simulink model "vinayquadcopter298"  (R2013b)
settings: Solver=ode45  StartTime=0.0  StopTime=10  RelTol=1e-3  EnableMultiTasking=on
values from neighbouring files (symbols this model uses):
  b = 3.13*10^(-5)    (= 3.13e-05)    [vinayparameters.m]
  d = 7.5*10^(-7)    (= 7.5e-07)    [vinayparameters.m]
  g = 9.81    [vinayparameters.m]
  Ix = 7.5*10^(-3)    (= 0.0075)    [vinayparameters.m]
  Iy = 7.5*10^(-3)    (= 0.0075)    [vinayparameters.m]
  Iz = 1.3*10^(-2)    (= 0.013)    [vinayparameters.m]
  Jr = 6.5*10^(-5)    (= 6.5e-05)    [vinayparameters.m]
  kdp = 0.4    [vinayparameters.m]
  kdps = 0.4    [vinayparameters.m]
  kdt = 0.4    [vinayparameters.m]
  kdz = 20    [vinayparameters.m]
  kpp = 0.8    [vinayparameters.m]
  kpps = 1    [vinayparameters.m]
  kpt = 1.2    [vinayparameters.m]
  kpz = 100    [vinayparameters.m]
  l = 0.23    [vinayparameters.m]
  m = 0.65    [vinayparameters.m]
libraries: simulink x7
settings Model: Creator=lcoelab  LastModifiedBy=VINAY
settings DataIOCC: SignalLoggingSaveFormat=ModelDataLogs
settings OptimizationCC: SimCompilerOptimization=off
settings DebuggingCC: UnderspecifiedInitializationDetection=Simplified  MergeDetectMultiDrivingBlocksExec=error  MultiTaskDSMMsg=warning  MultiTaskCondExecSysMsg=none  FcnCallInpInsideContextMsg=error  FrameProcessingCompatibilityMsg=error  LibraryContextMissingDiagnostic=warning  SFExecutionAtInitializationDiag=none
settings HardwareCC: ProdBitPerSizeT=32  ProdBitPerPtrDiffT=32
settings RTWCC: RTWCompilerOptimization=off
settings CodeAppCC: StateflowObjectComments=on
settings GRTTargetCC: TargetLangStandard=C89/C90 (ANSI)  CodeReplacementLibrary=None  CPPClassGenCompliant=on
settings ConfigComp: CovMetricSettings=dw  CovHtmlReporting=on  CovSaveCumulativeToWorkspaceVar=on  CovSaveSingleToWorkspaceVar=on  CovExternalEMLEnable=off

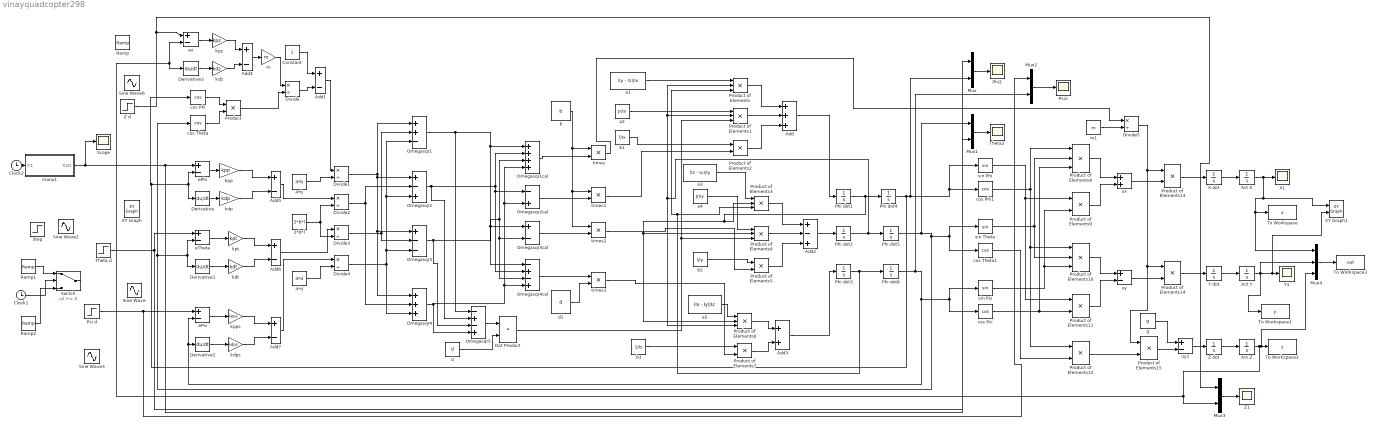
== system vinayquadcopter298 ==
  2*b*l : Constant  Value=2*b*l
  4*b : Constant  Value=4*b
  4*d : Constant  Value=4*d
  Act X : Integrator
  Act Y : Integrator
  Act Z : Integrator
  Add : Sum  Inputs=+++
  Add{1,4..7} (5 alike) : Sum  Inputs=+-
  Add2 : Sum  Inputs=+-+
  Add3 : Sum
  Clock1 : Clock
  Clock2 : Clock
  Constant : Constant
  Derivative{,1..3} (4 alike) : Derivative
  Divide{,1..5} (6 alike) : Product  Inputs=*/
  Dot Product : DotProduct  InputSameDT=on  OutDataTypeStr=Inherit: Inherit via internal rule
  Mux{,1..3} (4 alike) : Mux  Inputs=2
  Mux4 : Mux  Inputs=3
  Omegasqr1 : Sum  Inputs=++-
  Omegasqr1cal : Sum  Inputs=++++
  Omegasqr2 : Sum  Inputs=+-+
  Omegasqr2cal : Sum  Inputs=-+
  Omegasqr3 : Sum  Inputs=+--
  Omegasqr3cal : Sum  Inputs=+-
  Omegasqr4 : Sum  Inputs=+++
  Omegasqr4cal : Sum  Inputs=-+-+
  Omegasqr5 : Sum  Inputs=-+-+
  Phi dot1 : Integrator
  Phi dot{2..6} (5 alike) : Integrator  ZeroCross=off
  Phi2 : Scope
  Product : Product  RndMeth=Zero
  Product of Elements{,1,3..4,6,8,10} (7 alike) : Product  Inputs=3
  Product of Elements{2,5,7,9,11..15} (9 alike) : Product
  Psi d : Step  Time=0  After=0  SampleTime=0
  Psi2 : Scope
  Ramp : simulink/Sources/Ramp  slope=1  start=0  X0=0
  Ramp1 : simulink/Sources/Ramp  slope=0.1  start=0  X0=0
  Ramp2 : simulink/Sources/Ramp  slope=-0.1  start=0  X0=0
  Scope : Scope
  Sine Wave : Sin  Amplitude=10  Frequency=0.005*(2*pi)  Phase=pi/2  SampleTime=0
  Sine Wave2 : Sin  Amplitude=10  Frequency=0.005*(2*pi)  SampleTime=0
  Sine Wave3 : Sin  SampleTime=0
  Sine Wave6 : Sin  Amplitude=0  Frequency=0  SampleTime=0
  Step : Step  Time=0  After=5  SampleTime=0
  Switch : Switch  Threshold=4  SaturateOnIntegerOverflow=off  InputSameDT=off
  Theta d : Step  Time=0  After=0  SampleTime=0
  Theta2 : Scope
  To Workspace : ToWorkspace  VariableName=x  SampleTime=-1
  To Workspace1 : ToWorkspace  VariableName=y  SampleTime=-1
  To Workspace2 : ToWorkspace  VariableName=z  SampleTime=-1
  To Workspace3 : ToWorkspace  VariableName=out  SampleTime=-1  SaveFormat=Timeseries
  X dot : Integrator
  X1 : Scope
  XY Graph : simulink/Sinks/XY Graph  xmin=-20  xmax=20  ymin=-20  ymax=20  st=-1
  XY Graph1 : simulink/Sinks/XY Graph  xmin=-100  xmax=100  ymin=-100  ymax=100  st=-1
  Y dot : Integrator
  Y1 : Scope
  Z d : Step  Time=0  After=5  SampleTime=0
  Z dot : Integrator
  Z1 : Scope
  a1 : Constant  Value=(Iy - Iz)/Ix
  a2 : Constant  Value=Jr/Ix
  a3 : Constant  Value=(Iz - Ix)/Iy
  a4 : Constant  Value=Jr/Iy
  a5 : Constant  Value=(Ix - Iy)/Iz
  b : Constant  Value=b
  b1 : Constant  Value=l/Ix
  b2 : Constant  Value=l/Iy
  b3 : Constant  Value=1/Iz
  cos Phi : Trigonometry  Operator=cos
  cos Phi1 : Trigonometry  Operator=cos
  cos Psi : Trigonometry  Operator=cos
  cos Theta : Trigonometry  Operator=cos
  cos Theta1 : Trigonometry  Operator=cos
  d : Constant  Value=d
  d1 : Constant  Value=d
  ePhi : Sum  Inputs=+-
  ePsi : Sum  Inputs=+-
  eTheta : Sum  Inputs=+-
  ez : Sum  Inputs=+-
  g : Constant  Value=g
  kdp : Gain  Gain=kdp
  kdps : Gain  Gain=kdps
  kdt : Gain  Gain=kdt
  kdz : Gain  Gain=kdz
  kpp : Gain  Gain=kpp
  kpps : Gain  Gain=kpps
  kpt : Gain  Gain=kpt
  kpz : Gain  Gain=kpz
  m : Gain  Gain=m
  m1 : Constant  Value=m
  manu1 : Subsystem  TreatAsAtomicUnit=on
  sin Phi : Trigonometry
  sin Psi : Trigonometry
  sin Theta : Trigonometry
  times{,1..3} (4 alike) : Product  Inputs=**
  ux : Sum
  uy : Sum  Inputs=+-
  uy1 : Sum  Inputs=+-
  wires:
  Phi dot4/1 -> sin Phi/1, cos Phi1/1, Mux/2, cos Phi/1, Derivative/1, ePhi/2
  Phi dot5/1 -> cos Theta/1, Derivative1/1, eTheta/2, cos Theta1/1, sin Theta/1, Mux1/1
  Phi dot6/1 -> ePsi/2, Derivative2/1, sin Psi/1, cos Psi/1, Mux2/2
  ePhi/1 -> kpp/1
  Derivative/1 -> kdp/1
  eTheta/1 -> kpt/1
  Derivative1/1 -> kdt/1
  ePsi/1 -> kpps/1
  Derivative2/1 -> kdps/1
  ez/1 -> kpz/1
  Derivative3/1 -> kdz/1
  kpz/1 -> Add4/1
  kdz/1 -> Add4/2
  kpp/1 -> Add5/1
  kdp/1 -> Add5/2
  kpt/1 -> Add6/1
  kdt/1 -> Add6/2
  kpps/1 -> Add7/1
  kdps/1 -> Add7/2
  cos Phi/1 -> Product/1
  cos Theta/1 -> Product/2
  Add4/1 -> m/1
  m/1 -> Divide/1
  Product/1 -> Divide/2
  Constant/1 -> Add1/1
  Divide/1 -> Add1/2
  Add1/1 -> Divide1/1
  4*b/1 -> Divide1/2
  Add5/1 -> Divide2/1
  2*b*l/1 -> Divide2/2, Divide3/2
  Add6/1 -> Divide3/1
  Add7/1 -> Divide4/1
  4*d/1 -> Divide4/2
  Divide1/1 -> Omegasqr1/1, Omegasqr2/1, Omegasqr3/1, Omegasqr4/1
  Divide3/1 -> Omegasqr1/2, Omegasqr3/2
  Divide4/1 -> Omegasqr1/3, Omegasqr2/3, Omegasqr3/3, Omegasqr4/3
  Divide2/1 -> Omegasqr2/2, Omegasqr4/2
  Omegasqr1/1 -> Omegasqr5/1, Omegasqr3cal/1, Omegasqr4cal/1, Omegasqr1cal/1
  Omegasqr2/1 -> Omegasqr5/2, Omegasqr2cal/1, Omegasqr4cal/2, Omegasqr1cal/2
  Omegasqr3/1 -> Omegasqr5/3, Omegasqr1cal/3, Omegasqr3cal/2, Omegasqr4cal/3
  Omegasqr4/1 -> Omegasqr5/4, Omegasqr1cal/4, Omegasqr2cal/2, Omegasqr4cal/4
  Omegasqr5/1 -> Dot Product/1
  d/1 -> Dot Product/2
  b/1 -> times/1, times1/1, times2/1
  Omegasqr1cal/1 -> times/2
  Omegasqr2cal/1 -> times1/2
  Omegasqr3cal/1 -> times2/2
  Omegasqr4cal/1 -> times3/1
  d1/1 -> times3/2
  Product of Elements/1 -> Add/1
  Product of Elements1/1 -> Add/2
  Product of Elements2/1 -> Add/3
  a1/1 -> Product of Elements/1
  Phi dot2/1 -> Product of Elements/2, Product of Elements1/2, Product of Elements6/3, Phi dot5/1
  Phi dot3/1 -> Product of Elements/3, Product of Elements3/3, Phi dot6/1
  a2/1 -> Product of Elements1/1
  b1/1 -> Product of Elements2/1
  times1/1 -> Product of Elements2/2
  Dot Product/1 -> Product of Elements1/3, Product of Elements4/3
  Product of Elements3/1 -> Add2/1
  Product of Elements4/1 -> Add2/2
  Product of Elements5/1 -> Add2/3
  a3/1 -> Product of Elements3/1
  a4/1 -> Product of Elements4/1
  b2/1 -> Product of Elements5/1
  times2/1 -> Product of Elements5/2
  Phi dot1/1 -> Product of Elements6/2, Product of Elements4/2, Product of Elements3/2, Phi dot4/1
  Product of Elements6/1 -> Add3/1
  Product of Elements7/1 -> Add3/2
  times3/1 -> Product of Elements7/2
  b3/1 -> Product of Elements7/1
  a5/1 -> Product of Elements6/1
  Add/1 -> Phi dot1/1
  Add2/1 -> Phi dot2/1
  Add3/1 -> Phi dot3/1
  sin Theta/1 -> Product of Elements8/2, Product of Elements10/2
  cos Psi/1 -> Product of Elements8/3, Product of Elements11/2
  cos Phi1/1 -> Product of Elements8/1, Product of Elements10/1, Product of Elements12/1
  sin Phi/1 -> Product of Elements9/1, Product of Elements11/1
  sin Psi/1 -> Product of Elements9/2, Product of Elements10/3
  Product of Elements8/1 -> ux/1
  Product of Elements9/1 -> ux/2
  ux/1 -> Product of Elements13/2
  Product of Elements10/1 -> uy/1
  Product of Elements11/1 -> uy/2
  uy/1 -> Product of Elements14/2
  cos Theta1/1 -> Product of Elements12/2
  Product of Elements12/1 -> Product of Elements15/2
  times/1 -> Divide5/1
  m1/1 -> Divide5/2
  Divide5/1 -> Product of Elements13/1, Product of Elements14/1, Product of Elements15/1
  Product of Elements13/1 -> X dot/1
  Product of Elements14/1 -> Y dot/1
  uy1/1 -> Z dot/1
  Product of Elements15/1 -> uy1/2
  g/1 -> uy1/1
  X dot/1 -> Act X/1
  Y dot/1 -> Act Y/1
  Z dot/1 -> Act Z/1
  Act Y/1 -> Mux4/2, XY Graph1/2, Y1/1, To Workspace1/1
  Mux/1 -> Phi2/1
  Mux1/1 -> Theta2/1
  Theta d/1 -> Mux1/2, eTheta/1
  Mux2/1 -> Psi2/1
  Act Z/1 -> Mux4/3, To Workspace2/1, ez/2, Derivative3/1, Mux3/2
  Psi d/1 -> Mux2/1, ePsi/1
  Act X/1 -> Mux4/1, To Workspace/1, XY Graph1/1, X1/1
  Mux3/1 -> Z1/1
  Z d/1 -> Mux3/1, ez/1
  Mux4/1 -> To Workspace3/1
  manu1/1(Out1) -> Mux/1, ePhi/1, Scope/1
  Clock2/1 -> manu1/1(In1)
  Ramp1/1 -> Switch/1
  Clock1/1 -> Switch/2
  Ramp2/1 -> Switch/3

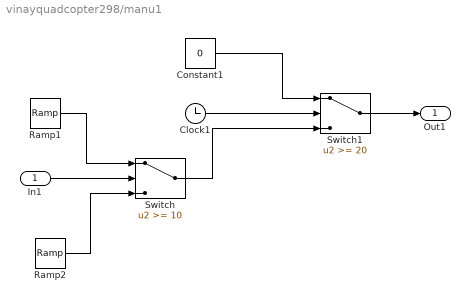
== system vinayquadcopter298/manu1 ==
  In1 : Inport
  Clock1 : Clock
  Constant1 : Constant  Value=0
  Ramp1 : simulink/Sources/Ramp  slope=0.5  start=0  X0=0
  Ramp2 : simulink/Sources/Ramp  slope=-0.5  start=0  X0=0
  Switch : Switch  Threshold=10  SaturateOnIntegerOverflow=off  InputSameDT=off
  Switch1 : Switch  Threshold=20  SaturateOnIntegerOverflow=off  InputSameDT=off
  Out1 : Outport
  wires:
  Ramp2/1 -> Switch/3
  Ramp1/1 -> Switch/1
  Switch/1 -> Switch1/3
  Clock1/1 -> Switch1/2
  Constant1/1 -> Switch1/1
  Switch1/1 -> Out1/1
  In1/1 -> Switch/2
